simulink model "Actuator2"  (R2025b)
settings: Solver=VariableStepAuto  StartTime=0.0  StopTime=10.0  RelTol=1e-3
settings Model: Creator=mikol  LastModifiedBy=mikol

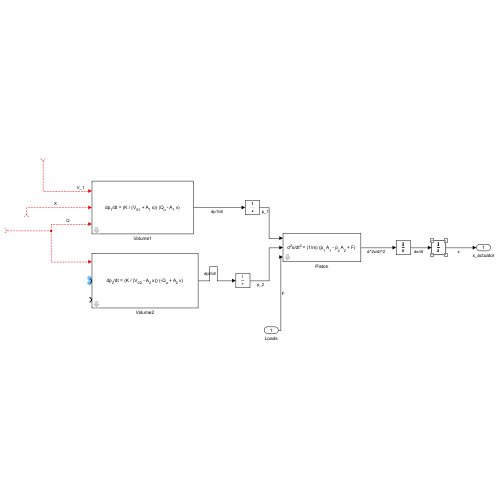
[thumbnail: Simulink's stored preview of the top-level diagram]
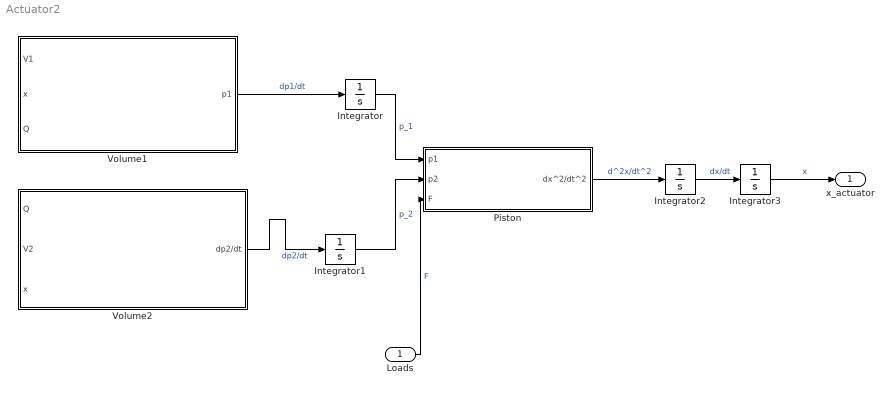
== system Actuator2 ==
  Loads : Inport
  Integrator{,1..3} (4 alike) : Integrator
  Piston : Subsystem
      mask Display: disp('d^2x/dt^2 = (1/m) (p_1 A_1 - p_2 A_2 + F)', 'texmode', 'on')
  Volume1 : Subsystem
      mask Display: disp('dp_1/dt = (K / (V_{01} + A_1 x)) (Q_u - A_1 v)', 'texmode', 'on')
  Volume2 : Subsystem
      mask Display: disp('dp_2/dt = (K / (V_{02} - A_2 x)) (-Q_u + A_2 v)', 'texmode', 'on')
  x_actuator : Outport
  wires:
  ? -> Volume1/3(Q), Volume2/1(Q)  "Q"
  ? -> Volume1/1(V1)  "V_1"
  ? -> Volume1/2(x)  "X"
  Volume1/1(p1) -> Integrator/1  "dp1/dt"
  Volume2/1(dp2/dt) -> Integrator1/1  "dp2/dt"
  Integrator/1 -> Piston/1(p1)  "p_1"
  Integrator1/1 -> Piston/2(p2)  "p_2"
  Piston/1(dx^2/dt^2) -> Integrator2/1  "d^2x/dt^2"
  Integrator2/1 -> Integrator3/1  "dx/dt"
  Integrator3/1 -> x_actuator/1  "x"
  Loads/1 -> Piston/3(F)  "F"

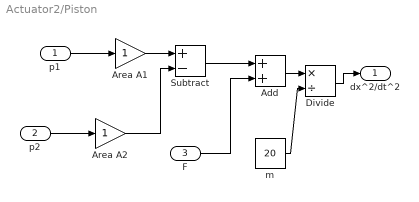
== system Actuator2/Piston ==
  p1 : Inport
  p2 : Inport  Port=2
  F : Inport  Port=3
  Add : Sum
  Area A1 : Gain
  Area A2 : Gain
  Divide : Product  Inputs=*/
  Subtract : Sum  Inputs=+-
  m : Constant  Value=20
  dx^2/dt^2 : Outport
  wires:
  p2/1 -> Area A2/1
  p1/1 -> Area A1/1
  Area A1/1 -> Subtract/1
  Area A2/1 -> Subtract/2
  Subtract/1 -> Add/1
  F/1 -> Add/2
  Add/1 -> Divide/1
  m/1 -> Divide/2
  Divide/1 -> dx^2/dt^2/1

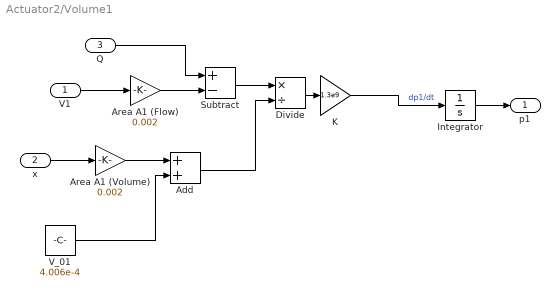
== system Actuator2/Volume1 ==
  V1 : Inport
  x : Inport  Port=2
  Q : Inport  Port=3
  Add : Sum
  Area A1 (Flow) : Gain  Gain=0.002
  Area A1 (Volume) : Gain  Gain=0.002
  Divide : Product  Inputs=*/
  Integrator : Integrator
  K : Gain  Gain=1.3e9
  Subtract : Sum  Inputs=+-
  V_01 : Constant  Value=4.006e-4
  p1 : Outport
  wires:
  Integrator/1 -> p1/1
  K/1 -> Integrator/1  "dp1/dt"
  V1/1 -> Area A1 (Flow)/1
  Area A1 (Flow)/1 -> Subtract/2
  Q/1 -> Subtract/1
  Subtract/1 -> Divide/1
  Divide/1 -> K/1
  x/1 -> Area A1 (Volume)/1
  Area A1 (Volume)/1 -> Add/1
  V_01/1 -> Add/2
  Add/1 -> Divide/2

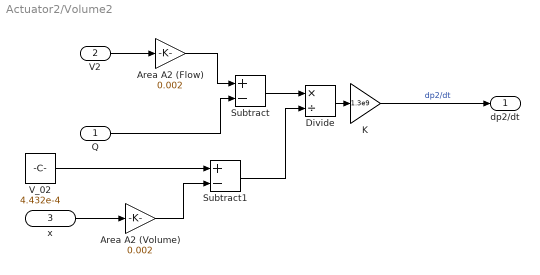
== system Actuator2/Volume2 ==
  Q : Inport
  V2 : Inport  Port=2
  x : Inport  Port=3
  Area A2 (Flow) : Gain  Gain=0.002
  Area A2 (Volume) : Gain  Gain=0.002
  Divide : Product  Inputs=*/
  K : Gain  Gain=1.3e9
  Subtract : Sum  Inputs=+-
  Subtract1 : Sum  Inputs=+-
  V_02 : Constant  Value=4.432e-4
  dp2/dt : Outport
  wires:
  Subtract1/1 -> Divide/2
  K/1 -> dp2/dt/1  "dp2/dt"
  Area A2 (Flow)/1 -> Subtract/1
  Divide/1 -> K/1
  V2/1 -> Area A2 (Flow)/1
  x/1 -> Area A2 (Volume)/1
  Subtract/1 -> Divide/1
  V_02/1 -> Subtract1/1
  Q/1 -> Subtract/2
  Area A2 (Volume)/1 -> Subtract1/2
